simulink model "StateflowBlock"  (R2024b)
settings: Solver=FixedStepDiscrete  StartTime=0.0  StopTime=Inf  FixedStep=0.1  RelTol=1e-3
settings Model: TunableVars=kp,PWMsl_l,PWMsl_r,PWMsr_l,PWMsr_r  TunableVarsStorageClass=Auto,Auto,Auto,Auto,Auto  TunableVarsTypeQualifier=,,,,  Creator=omars  LastModifiedBy=eggyg
settings DataIOCC: ReturnWorkspaceOutputs=off
settings OptimizationCC: EnhancedBackFolding=on  PassReuseOutputArgsAs=Individual arguments  ZeroExternalMemoryAtStartup=off  ZeroInternalMemoryAtStartup=off  OptimizeBlockOrder=speed  DifferentSizesBufferReuse=on  OptimizationCustomize=off  EfficientTunableParamExpr=on
settings DebuggingCC: ParameterTunabilityLossMsg=error
settings SFSimCC: MATLABDynamicMemAlloc=off
settings RTWCC: Description=Embedded Coder  SystemTargetFile=ert.tlc  GenCodeOnly=on  TemplateMakefile=ert_default_tmf  GPUComputeCapability=3.5
settings CodeAppCC: ForceParamTrailComments=on  IgnoreCustomStorageClasses=off  OperatorAnnotations=on  SimulinkDataObjDesc=on  SFDataObjDesc=on  InsertBlockDesc=on
settings ERTTargetCC: TargetLangStandard=C99 (ISO)  SupportVariableSizeSignals=on  InlinedParameterPlacement=Hierarchical  ERTCustomFileTemplate=example_file_process.tlc  DynamicArrayContainerType=coder::array

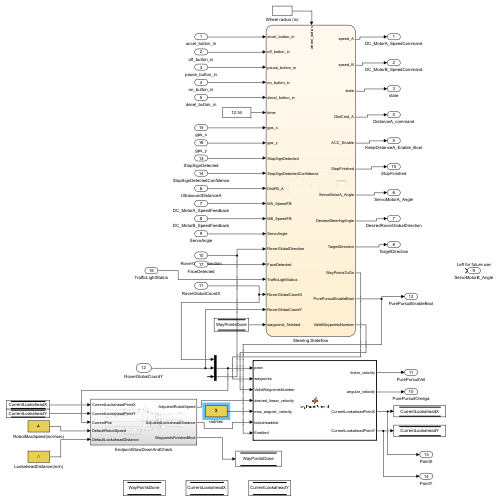
[thumbnail: Simulink's stored preview of the top-level diagram]
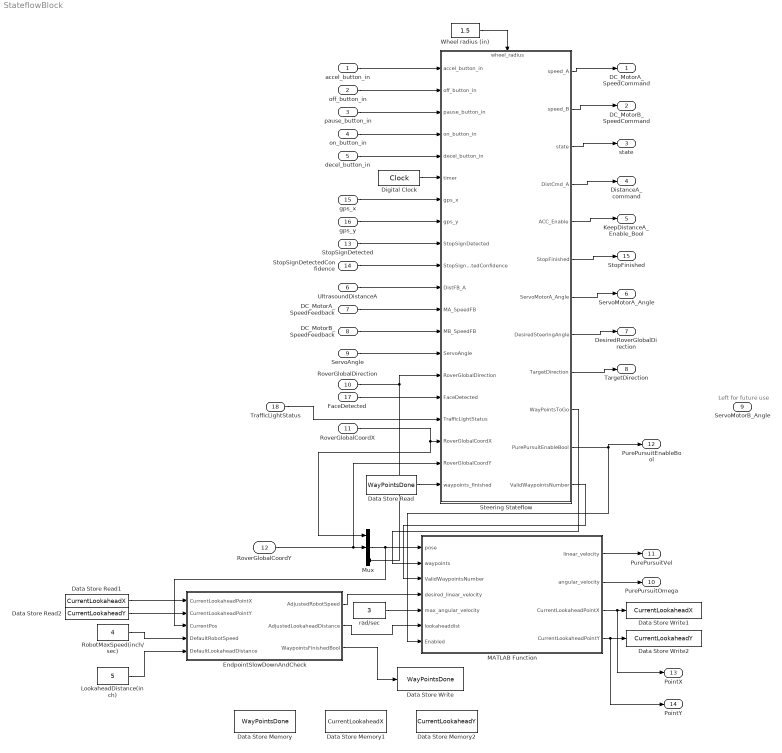
== system StateflowBlock ==
  note: Left for future use
  accel_button_in : Inport
  off_button_in : Inport  Port=2
  pause_button_in : Inport  Port=3
  on_button_in : Inport  Port=4
  decel_button_in : Inport  Port=5
  UltrasoundDistanceA : Inport  Port=6
  DC_MotorA_SpeedFeedback : Inport  Port=7
  DC_MotorB_SpeedFeedback : Inport  Port=8
  ServoAngle : Inport  Port=9
  RoverGlobalDirection : Inport  Port=10
  RoverGlobalCoordX : Inport  Port=11
  RoverGlobalCoordY : Inport  Port=12
  StopSignDetected : Inport  Port=13
  StopSignDetectedConfidence : Inport  Port=14
  gps_x : Inport  Port=15
  gps_y : Inport  Port=16
  FaceDetected : Inport  Port=17
  TrafficLightStatus : Inport  Port=18
  Data Store Memory : DataStoreMemory  DataStoreName=WayPointsDone  WriteAfterWriteMsg=warning  ShowAdditionalParam=off
  Data Store Memory1 : DataStoreMemory  DataStoreName=CurrentLookaheadX  WriteAfterWriteMsg=warning  ShowAdditionalParam=off
  Data Store Memory2 : DataStoreMemory  DataStoreName=CurrentLookaheadY  WriteAfterWriteMsg=warning  ShowAdditionalParam=off
  Data Store Read : DataStoreRead  DataStoreName=WayPointsDone  IndexOptions=Index vector (dialog)  Indices=1  OutputSizes=1
  Data Store Read1 : DataStoreRead  DataStoreName=CurrentLookaheadX  IndexOptions=Index vector (dialog)  Indices=1  OutputSizes=1
  Data Store Read2 : DataStoreRead  DataStoreName=CurrentLookaheadY  IndexOptions=Index vector (dialog)  Indices=1  OutputSizes=1
  Data Store Write : DataStoreWrite  DataStoreName=WayPointsDone  IndexOptions=Index vector (dialog)  Indices=1  OutputSizes=1
  Data Store Write1 : DataStoreWrite  DataStoreName=CurrentLookaheadX  IndexOptions=Index vector (dialog)  Indices=1  OutputSizes=1
  Data Store Write2 : DataStoreWrite  DataStoreName=CurrentLookaheadY  IndexOptions=Index vector (dialog)  Indices=1  OutputSizes=1
  Digital Clock : DigitalClock  SampleTime=0.1
  EndpointSlowDownAndCheck : Subsystem
  LookaheadDistance(inch) : Constant  Value=5
  MATLAB Function : MATLAB Function  TreatAsAtomicUnit=on
  Mux : Mux  Inputs=3
  RobotMaxSpeed(inch/sec) : Constant  Value=4
  Steering Stateflow : Stateflow chart  TreatAsAtomicUnit=on
      settings: PortSchema="{\"entries\":[{\"content\":{\"sides\":[{\"content\":{\"connectorIds\":[\"In3\",\"In4\",\"In6\",\"In11\",\"In21\",\"In5\",\"In7\",\"In8\",\"In9\",\"In10\",\"In1\",\"In12\",\"In13\",\"In14\",\"In15\",\"In18\",\"In17\",\"In16\",\"In19\",\"In20\"]},\"type\":\"ConnectorPlacement.EquallySpacedRectSide\",\"uuid\":\"80dcc8d6-aa19-4329-80f2-43be3f76ecea\"},{\"content\":{\"connectorIds\":[\"Out2\",\"Out3\",\"Out5\",\"Out4\",\"Out1\",\"Out6\",\"Out7\",\"Out8\",\"Out9\",\"Out10\",\"Out11\",\"Out12\"],\"side\":\"RIGHT\"},\"type\":\"ConnectorPlacement.EquallySpacedRectSide\",\"uuid\":\"4e6e0fce-41ed-43d9-af05-514bba8f8dbd\"},{\"content\":{\"connectorIds\":[\"In2\"],\"side\":\"TOP\"},\"type\":\"ConnectorPlacement.EquallySpacedRectSide\",\"uuid\":\"7ace72f0-dafc-45ef-b347-5f7d59858afe\"},{\"content\":{\"side\":\"BOTTOM\"},\"type\":\"ConnectorPlacement.EquallySpacedRectSide\",\"uuid\":\"573fd0e0-7faf-456f-ae2d-765ad0ec4cd5\"}]},\"type\":\"ConnectorPlacement.EquallySpacedConnector\",\"uuid\":\"0e6ea89e-5511-46b0-968b-5e141f0ce0a1\"}],\"packageUris\":[\"http://schema.mathworks.com/mf0/Connector/R2020b\"],\"version\":\"1.0\"}"
  Wheel radius (in) : Constant  Value=1.5
  rad/sec : Constant  Value=3
  DC_MotorA_SpeedCommand : Outport
  DC_MotorB_SpeedCommand : Outport  Port=2
  state : Outport  Port=3
  DistanceA_command : Outport  Port=4
  KeepDistanceA_Enable_Bool : Outport  Port=5
  ServoMotorA_Angle : Outport  Port=6
  DesiredRoverGlobalDirection : Outport  Port=7
  TargetDirection : Outport  Port=8
  ServoMotorB_Angle : Outport  Port=9
  PurePursuitOmega : Outport  Port=10
  PurePursuitVel : Outport  Port=11
  PurePursuitEnableBool : Outport  Port=12
  PointX : Outport  Port=13
  PointY : Outport  Port=14
  StopFinished : Outport  Port=15
  wires:
  pause_button_in/1 -> Steering Stateflow/6(pause_button_in)
  Steering Stateflow/3(speed_B) -> DC_MotorB_SpeedCommand/1
  Steering Stateflow/5(state) -> state/1
  Steering Stateflow/2(speed_A) -> DC_MotorA_SpeedCommand/1
  off_button_in/1 -> Steering Stateflow/4(off_button_in)
  accel_button_in/1 -> Steering Stateflow/3(accel_button_in)
  decel_button_in/1 -> Steering Stateflow/21(decel_button_in)
  on_button_in/1 -> Steering Stateflow/11(on_button_in)
  Wheel radius (in)/1 -> Steering Stateflow/2(wheel_radius)
  Steering Stateflow/4(DistCmd_A) -> DistanceA_command/1
  Steering Stateflow/1(ACC_Enable) -> KeepDistanceA_Enable_Bool/1
  UltrasoundDistanceA/1 -> Steering Stateflow/1(DistFB_A)
  DC_MotorB_SpeedFeedback/1 -> Steering Stateflow/13(MB_SpeedFB)
  DC_MotorA_SpeedFeedback/1 -> Steering Stateflow/12(MA_SpeedFB)
  Steering Stateflow/7(ServoMotorA_Angle) -> ServoMotorA_Angle/1
  ServoAngle/1 -> Steering Stateflow/14(ServoAngle)
  Steering Stateflow/8(DesiredSteeringAngle) -> DesiredRoverGlobalDirection/1
  RoverGlobalDirection/1 -> Mux/3, Steering Stateflow/15(RoverGlobalDirection)
  Steering Stateflow/9(TargetDirection) -> TargetDirection/1
  RoverGlobalCoordX/1 -> Mux/1, Steering Stateflow/16(RoverGlobalCoordX)
  RoverGlobalCoordY/1 -> Steering Stateflow/19(RoverGlobalCoordY), Mux/2
  Mux/1 -> EndpointSlowDownAndCheck/3(CurrentPos), MATLAB Function/1(pose)
  MATLAB Function/2(angular_velocity) -> PurePursuitOmega/1
  MATLAB Function/1(linear_velocity) -> PurePursuitVel/1
  Steering Stateflow/10(WayPointsToGo) -> MATLAB Function/2(waypoints)
  Steering Stateflow/11(PurePursuitEnableBool) -> PurePursuitEnableBool/1, MATLAB Function/7(Enabled)
  Data Store Read/1 -> Steering Stateflow/20(waypoints_finished)
  Steering Stateflow/12(ValidWaypointsNumber) -> MATLAB Function/3(ValidWaypointsNumber)
  rad/sec/1 -> MATLAB Function/5(max_angular_velocity)
  RobotMaxSpeed(inch/sec)/1 -> EndpointSlowDownAndCheck/4(DefaultRobotSpeed)
  LookaheadDistance(inch)/1 -> EndpointSlowDownAndCheck/5(DefaultLookaheadDistance)
  EndpointSlowDownAndCheck/1(AdjustedRobotSpeed) -> MATLAB Function/4(desired_linear_velocity)
  EndpointSlowDownAndCheck/2(AdjustedLookaheadDistance) -> MATLAB Function/6(lookaheaddist)
  MATLAB Function/3(CurrentLookaheadPointX) -> PointX/1, Data Store Write1/1
  MATLAB Function/4(CurrentLookaheadPointY) -> PointY/1, Data Store Write2/1
  Data Store Read1/1 -> EndpointSlowDownAndCheck/1(CurrentLookaheadPointX)
  Data Store Read2/1 -> EndpointSlowDownAndCheck/2(CurrentLookaheadPointY)
  EndpointSlowDownAndCheck/3(WaypointsFinishedBool) -> Data Store Write/1
  Digital Clock/1 -> Steering Stateflow/5(timer)
  StopSignDetected/1 -> Steering Stateflow/9(StopSignDetected)
  Steering Stateflow/6(StopFinished) -> StopFinished/1
  StopSignDetectedConfidence/1 -> Steering Stateflow/10(StopSignDetectedConfidence)
  gps_x/1 -> Steering Stateflow/7(gps_x)
  gps_y/1 -> Steering Stateflow/8(gps_y)
  FaceDetected/1 -> Steering Stateflow/18(FaceDetected)
  TrafficLightStatus/1 -> Steering Stateflow/17(TrafficLightStatus)

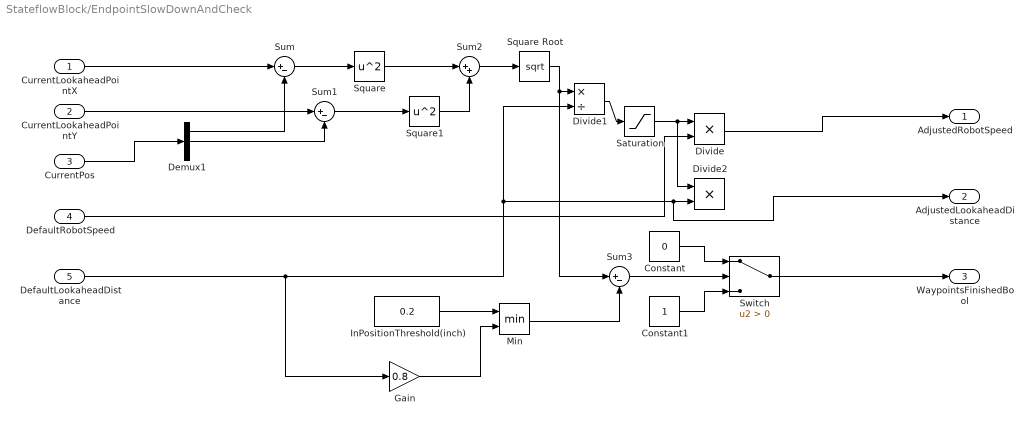
== system StateflowBlock/EndpointSlowDownAndCheck ==
  CurrentLookaheadPointX : Inport
  CurrentLookaheadPointY : Inport  Port=2
  CurrentPos : Inport  Port=3
  DefaultRobotSpeed : Inport  Port=4
  DefaultLookaheadDistance : Inport  Port=5
  Constant : Constant  Value=0
  Constant1 : Constant
  Demux1 : Demux  Outputs=3
  Divide : Product  Inputs=**
  Divide1 : Product  Inputs=*/
  Divide2 : Product  Inputs=**
  Gain : Gain  Gain=0.8
  InPositionThreshold(inch) : Constant  Value=0.2
  Min : MinMax  Inputs=2
  Saturation : Saturate  UpperLimit=1  LowerLimit=-1
  Square : Math  Operator=square
  Square Root : Sqrt
  Square1 : Math  Operator=square
  Sum : Sum  Inputs=|+-
  Sum1 : Sum  Inputs=|+-
  Sum2 : Sum  Inputs=|++
  Sum3 : Sum  Inputs=|+-
  Switch : Switch  Criteria=u2 > Threshold  SaturateOnIntegerOverflow=off  InputSameDT=off
  AdjustedRobotSpeed : Outport
  AdjustedLookaheadDistance : Outport  Port=2
  WaypointsFinishedBool : Outport  Port=3
  wires:
  CurrentPos/1 -> Demux1/1
  CurrentLookaheadPointX/1 -> Sum/1
  Demux1/1 -> Sum/2
  CurrentLookaheadPointY/1 -> Sum1/1
  Demux1/2 -> Sum1/2
  Sum/1 -> Square/1
  Sum1/1 -> Square1/1
  Square/1 -> Sum2/1
  Square1/1 -> Sum2/2
  Sum2/1 -> Square Root/1
  Saturation/1 -> Divide2/1, Divide/1
  DefaultRobotSpeed/1 -> Divide/2
  Divide/1 -> AdjustedRobotSpeed/1
  Square Root/1 -> Sum3/1, Divide1/1
  Divide1/1 -> Saturation/1
  DefaultLookaheadDistance/1 -> Gain/1, AdjustedLookaheadDistance/1, Divide2/2, Divide1/2
  Sum3/1 -> Switch/2
  Constant/1 -> Switch/1
  Constant1/1 -> Switch/3
  Switch/1 -> WaypointsFinishedBool/1
  InPositionThreshold(inch)/1 -> Min/1
  Min/1 -> Sum3/2
  Gain/1 -> Min/2

== matlab function StateflowBlock/MATLAB Function ==
  data: pose input double; linear_velocity output; waypoints input; ValidWaypointsNumber input; desired_linear_velocity input; max_angular_velocity input; lookaheaddist input; angular_velocity output; Enabled input; CurrentLookaheadPointX output; CurrentLookaheadPointY output
function [linear_velocity, angular_velocity, CurrentLookaheadPointX, CurrentLookaheadPointY] = MyPurePursuit(pose, waypoints, ValidWaypointsNumber, desired_linear_velocity, max_angular_velocity, lookaheaddist, Enabled)
% MyPurePursuit - Implements Pure Pursuit with internal waypoint index tracking


% Persistent variable to store current waypoint index
persistent waypoint_index;

CurrentLookaheadPointX = 99999; %Arbutual number
CurrentLookaheadPointY = 99999;
lookaheaddistSquare = lookaheaddist^2;
if(Enabled == 0)
    linear_velocity = 0;
    angular_velocity = 0; 
    waypoint_index = 1; % Standby for the next round
else

    % Initialize waypoint index on first call
    if isempty(waypoint_index)
        waypoint_index = 1;
    end

    % Extract robot state
    x = pose(1);
    y = pose(2);
    theta = pose(3);

    % Ensure index is within bounds
    if waypoint_index > ValidWaypointsNumber
        waypoint_index = ValidWaypointsNumber;
    end

    % Find the look-ahead point
    lookahead_point = [];
    if waypoint_index == ValidWaypointsNumber
        lookahead_point = waypoints(ValidWaypointsNumber,:);
        %IsTrackingFinalPoint = 1;
    else
        for i = waypoint_index:ValidWaypointsNumber
            %dist = sqrt((waypoints(i,1) - x)^2 + (waypoints(i,2) - y)^2);
            distSquare = (waypoints(i,1) - x)^2 + (waypoints(i,2) - y)^2; % Take out sqrt to reduce computation
            %if dist >= lookaheaddist
            if distSquare >= lookaheaddistSquare
                lookahead_point = waypoints(i, :);
                waypoint_index = i;  % Update to the next valid waypoint
                break;
            end
        end
    end
    % If no valid look-ahead point is found, stop the robot
    if isempty(lookahead_point)
        waypoint_index = ValidWaypointsNumber;
        lookahead_point = waypoints(ValidWaypointsNumber,:);
    end

    % Compute transformation to robot frame
    dx = lookahead_point(1) - x;
    dy = lookahead_point(2) - y;
    CurrentLookaheadPointX = lookahead_point(1);
    CurrentLookaheadPointY = lookahead_point(2);
    local_x = cos(theta) * dx + sin(theta) * dy;
    local_y = -sin(theta) * dx + cos(theta) * dy;
    distance2nextpointsquare = dx^2 + dy^2;

    % Compute curvature to target
    %curvature = 2 * local_y / (lookaheaddist^2);
    curvature = 2 * local_y / distance2nextpointsquare;

    % Compute angular velocity (omega)
    angular_velocity = desired_linear_velocity * curvature;

    % Apply angular velocity limit
    angular_velocity = max(min(angular_velocity, max_angular_velocity), -max_angular_velocity);

    % Set linear velocity
    linear_velocity = desired_linear_velocity;
    
end
end

== stateflow chart StateflowBlock/Steering Stateflow ==
  settings: updateMethod=DISCRETE  sampleTime=0.1
  state WayPointsGeneration
    %first straight
    WayPointsToGo(1,:) = [0 0];
    WayPointsToGo(2,:) = [45 0];
    WayPointsToGo(3,:) = [84 0];
    %first turn
    WayPointsToGo(4,:) = [96 0];
    WayPointsToGo(5,:) = [96 -4];
    WayPointsToGo(6,:) = [96 -12];
    WayPointsToGo(7,:) = [96 -20];
    WayPointsToGo(8,:) = [90 -20];
    WayPointsToGo(9,:) = [84 -20];
    %the hill
    WayPointsToGo(10,:) = [36 -20];
    WayPointsToGo(11,:) = [36 -36];
    ValidWaypointsNumber = 11;
    state = 11;
  state Test
    DistCmd_A = DistFB_A;
    DesiredSteeringAngle = RoverGlobalDirection + 360*5*pi/180;
    state = 21;
  state WaitngForTurning
    %DistCmd_A = DistFB_A;
    ACC_Enable = 1;
    state = 23;
  state OFF
    speed = 0
    speed_A = speed;
    speed_B = speed;
    state = 0;
    ACC_Enable = 0;
    DistCmd_A = 250;
    DesiredSteeringAngle = RoverGlobalDirection;
    ServoMotorA_Angle = 90;
    PurePursuitEnableBool = 0;
    WayPointsToGo = zeros(100,2);
  state WaitForGoing
    PurePursuitEnableBool = 1;
    state = 13;
  state Stop_for_5_seconds
    PurePursuitEnableBool = 0;
  note: Not used in this lab
  state WayPointsGeneration2
    WayPointsToGo(1,:) = [0 0];
    WayPointsToGo(2,:) = [3 0];
    WayPointsToGo(3,:) = [6 0];
    WayPointsToGo(4,:) = [9 0];
    WayPointsToGo(5,:) = [12 0];
    WayPointsToGo(6,:) = [15 0];
    WayPointsToGo(7,:) = [18 0];
    WayPointsToGo(8,:) = [21 0];
    WayPointsToGo(9,:) = [24 0];
    WayPointsToGo(10,:) = [24 3];
    WayPointsToGo(11,:) = [24 6];
    WayPointsToGo(12,:) = [24 9];
    WayPointsToGo(13,:) = [24 12];
    WayPointsToGo(14,:) = [24 15];
    WayPointsToGo(15,:) = [24 18];
    WayPointsToGo(16,:) = [24 21];
    WayPointsToGo(17,:) = [24 24];
    WayPointsToGo(18,:) = [21 24];
    WayPointsToGo(19,:) = [18 24];
    WayPointsToGo(20,:) = [15 24];
    WayPointsToGo(21,:) = [12 24];
    WayPointsToGo(22,:) = [9 24];
    WayPointsToGo(23,:) = [6 24];
    WayPointsToGo(24,:) = [3 24];
    WayPointsToGo(25,:) = [0 24];
    WayPointsToGo(26,:) = [0 21];
    WayPointsToGo(27,:) = [0 18];
    WayPointsToGo(28,:) = [0 15];
    WayPointsToGo(29,:) = [0 12];
    WayPointsToGo(30,:) = [0 9];
    WayPointsToGo(31,:) = [0 6];
    WayPointsToGo(32,:) = [0 3];
    WayPointsToGo(33,:) = [0 0];
    ValidWaypointsNumber = 33;
    state = 12;
  state SteeringToward
    state Initialize
      ServoASweepUpperLimit = 135; % Degree
      ServoASweepLowerLimit = 45; % Degree
      ServoASweepSpeed = 7;
      DistCmd_A = 30; % cm
      %
      ACC_Enable = 1;
      ServoASweepDirection = 1;
      ServoMotorA_Angle = ServoASweepLowerLimit;
      ServoAStopSweeping = 0;
      SweepingData = zeros(2,180);
      for i=1:180
      SweepingData(1,i) = 90;
      SweepingData(2,i) = 1500;
      end
      SweepingIndex = 0;
      %
      TurningAngleTrajectory = zeros(1,20);
      TurningAngleTrajectoryIndex = 1;
      for i=1:20
      TurningAngleTrajectory(i) = RoverGlobalDirection ;
      end
      state = 1;
    state Rurning
      DesiredSteeringAngle = TurningAngleTrajectory(TurningAngleTrajectoryIndex);
      if TurningAngleTrajectoryIndex < 20
      TurningAngleTrajectoryIndex = TurningAngleTrajectoryIndex + 1;
      end
      %TargetDirection = TargetGlobalAngle;
      state = 2;
    note: When angles are close, it means we reach the target angle
        | so we can proceed to do the next tracking
    state Scanning
      SweepingIndex = SweepingIndex + 1;
      SweepingData(1,SweepingIndex) = ServoMotorA_Angle;
      SweepingData(2,SweepingIndex) = DistFB_A;
      ServoMotorA_Angle = ServoMotorA_Angle + ServoASweepDirection*ServoASweepSpeed;
      if  ServoASweepDirection > 0
      if ServoMotorA_Angle >=ServoASweepUpperLimit
      ServoMotorA_Angle = ServoASweepUpperLimit;
      ServoAStopSweeping = 1;
      end
      else
      if ServoMotorA_Angle <=ServoASweepLowerLimit
      ServoMotorA_Angle = ServoASweepLowerLimit;
      ServoAStopSweeping = 1;
      end
      end
      state = 3;
    state TurningAngleTrajectoryPlaning1
      for i=1:20
      TurningAngleTrajectory(i) =TargetGlobalAngle;
      %No planning, just feeding the target angle directly
      end
      TurningAngleTrajectoryIndex = 1;
      state = 5;
    state GetObjectDirection
      ObjectDistance = 1500;
      ObjectDirection  = 90;
      for i=1:SweepingIndex
      TempDistance = SweepingData(2,i);
      if TempDistance<ObjectDistance
      ObjectDistance = TempDistance;
      ObjectDirection = SweepingData(1,i);
      end
      end
      ObjectDirection = ObjectDirection - ServoASweepDirection*ServoASweepSpeed*2;
      % This is for compasating the ultrasonic delay
      if ObjectDistance < 600  % There is an object in front
      TargetGlobalAngle = (ObjectDirection - 90)*pi/180 +RoverGlobalDirection;
      else
      TargetGlobalAngle = RoverGlobalDirection; % Don't turn
      end
      TargetDirection = ObjectDirection;
      ServoAStopSweeping = 0;
      ServoASweepDirection = -1*ServoASweepDirection;
      SweepingIndex = 0;
      for i=1:180
      SweepingData(1,i) = 90;
      SweepingData(2,i) = 1500;
      end
      state = 4;
    Initialize -> Rurning
    TurningAngleTrajectoryPlaning1 -> Rurning
    Rurning -> Scanning : [abs(TargetGlobalAngle-RoverGlobalDirection) < 0.1]
    (default) -> Initialize
    Scanning -> GetObjectDirection : [ServoAStopSweeping > 0]
    GetObjectDirection -> TurningAngleTrajectoryPlaning1
  state WayPointsGeneration4
    WayPointsToGo(1,:) = [0 0];
    WayPointsToGo(2,:) = [10 0];
    WayPointsToGo(3,:) = [10 10];
    WayPointsToGo(4,:) = [0 10];
    WayPointsToGo(5,:) = [0 0];
    ValidWaypointsNumber = 5;
    state = 16;
  Test -> WaitngForTurning
  WaitngForTurning -> OFF : [abs(DesiredSteeringAngle-RoverGlobalDirection) < 0.02]
  OFF -> WayPointsGeneration [order 3] : [accel_button_in > 0]
  WayPointsGeneration -> WaitForGoing
  WaitForGoing -> OFF [order 1] : [waypoints_finished == 1]
  (default) -> OFF
  WaitForGoing -> Stop_for_5_seconds [order 2] : [StopSignDetected > 0 && StopSignDetectedConfidence > 0.9]
      | {StopFinished = 1;}
  OFF -> WayPointsGeneration2 [order 2] : [decel_button_in > 0]
  Stop_for_5_seconds -> WaitForGoing : [after(5, sec)]{StopFinished = 0;}
  SteeringToward -> OFF : [off_button_in > 0]
  OFF -> WayPointsGeneration4 [order 1] : [on_button_in > 0]
  WayPointsGeneration4 -> WaitForGoing
  WayPointsGeneration2 -> WaitForGoing
  data: DistFB_A input; ACC_Enable output; wheel_radius input; accel_button_in input boolean; off_button_in input boolean; timer input; speed_A output double; speed_B output double; DistCmd_A output; pause_button_in input boolean =500; gps_x input single; gps_y input single; StopSignDetected input int32; StopSignDetectedConfidence input; state output; StopFinished output; on_button_in input; MA_SpeedFB input; MB_SpeedFB input; ServoAngle input; RoverGlobalDirection input; RoverGlobalCoordX input; TrafficLightStatus input; FaceDetected input; RoverGlobalCoordY input; waypoints_finished input; decel_button_in input; speed local; ServoMotorA_Angle output; DesiredSteeringAngle output; i local; ObjectDirection local; ObjectDistance local; TempDistance local; TargetGlobalAngle local; TurningAngleTrajectory local; TurningAngleTrajectoryIndex local; TargetDirection output; ServoASweepDirection local; ServoASweepSpeed local; ServoASweepUpperLimit local; ServoASweepLowerLimit local; ServoAStopSweeping local; SweepingData local; SweepingIndex local; WayPointsToGo output; PurePursuitEnableBool output; ValidWaypointsNumber output; data local
